simulink model "longmendiao_3"  (R2022b)
settings: Solver=VariableStepAuto  StartTime=0.0  StopTime=20  RelTol=1e-3
settings Model: Creator=MasterMo  LastModifiedBy=47800
settings SolverCC: AlgebraicLoopSolver=TrustRegion
settings DebuggingCC: UnconnectedInputMsg=warning  UnconnectedOutputMsg=warning  UnconnectedLineMsg=warning  SFMachineParentedDataDiag=warning
settings ModelReferenceCC: EnableRefExpFcnMdlSchedulingChecks=on

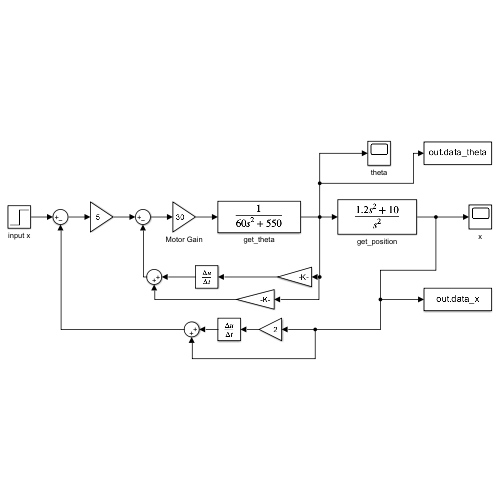
[thumbnail: Simulink's stored preview of the top-level diagram]
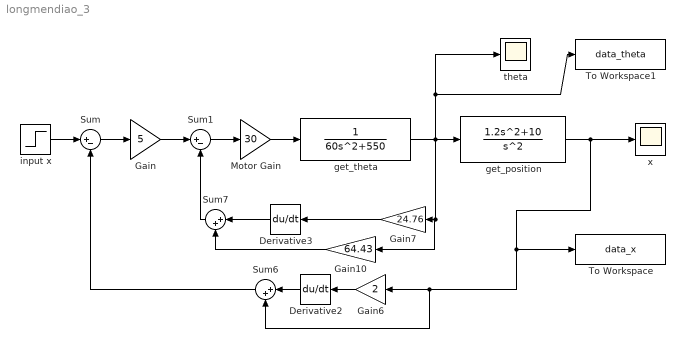
== system longmendiao_3 ==
  Derivative2 : Derivative
  Derivative3 : Derivative
  Gain : Gain  Gain=5
  Gain10 : Gain  Gain=64.43
  Gain6 : Gain  Gain=2
  Gain7 : Gain  Gain=24.76
  Motor Gain : Gain  Gain=30
  Sum : Sum  Inputs=|+-
  Sum1 : Sum  Inputs=|+-
  Sum6 : Sum  Inputs=|++
  Sum7 : Sum  Inputs=|++
  To Workspace : ToWorkspace  VariableName=data_x  SaveFormat=Structure With Time  SampleTime=-1
  To Workspace1 : ToWorkspace  VariableName=data_theta  SaveFormat=Structure With Time  SampleTime=-1
  get_position : TransferFcn  Numerator=[1.2 0 10]  Denominator=[1 0 0]
  get_theta : TransferFcn  Denominator=[60 0 550]
  input x : Step  After=8  SampleTime=0
  theta : Scope
  x : Scope
  wires:
  input x/1 -> Sum/1
  Motor Gain/1 -> get_theta/1
  Sum1/1 -> Motor Gain/1
  Gain/1 -> Sum1/1
  Sum/1 -> Gain/1
  Derivative2/1 -> Sum6/1
  Gain6/1 -> Derivative2/1
  get_position/1 -> Sum6/2, Gain6/1, To Workspace/1, x/1
  Sum6/1 -> Sum/2
  Gain7/1 -> Derivative3/1
  Sum7/1 -> Sum1/2
  Gain10/1 -> Sum7/2
  Derivative3/1 -> Sum7/1
  get_theta/1 -> Gain10/1, Gain7/1, To Workspace1/1, theta/1, get_position/1
